simulink model "pm4_motor"  (R2017a)
settings: Solver=VariableStepAuto  StartTime=0.0  StopTime=3.0  RelTol=1e-3
libraries: simulink x1
settings Model: Creator=robotica  LastModifiedBy=robotica

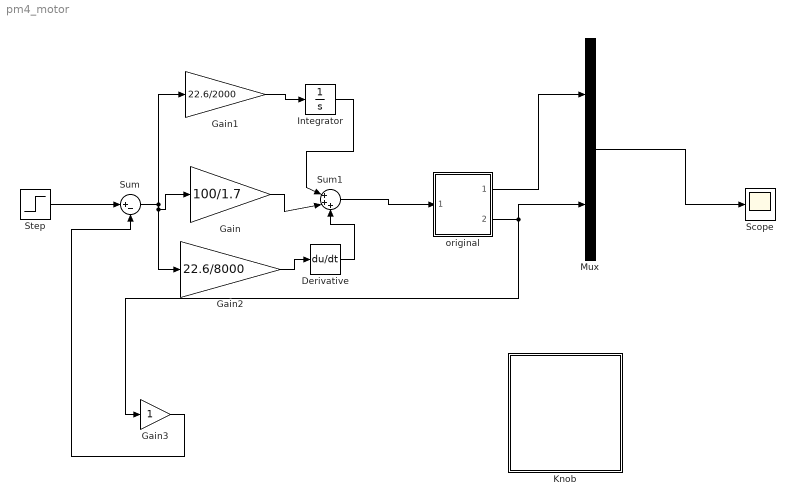
== system pm4_motor ==
  Derivative : Derivative
  Gain : Gain  Gain=100/1.7
  Gain1 : Gain  Gain=22.6/2000
  Gain2 : Gain  Gain=22.6/8000
  Gain3 : Gain
  Integrator : Integrator
  Knob : Subsystem  DialogController=hmiCreateDDGDialog  IsWebBlock=on  mask(MWDashboardBlock){webBlockId=eb4c633d-9a67-487d-a5e6-ad79ce51d936, webBlockType=continuousknob, ShowInLibBrowser=on, ShowInitialText=on, HMISrcModelName=pm4_motor}
      mask prompts: webBlockId "WebBlock Id"; webBlockType "WebBlock Type"; HMISrcModelName "Source Model"
      mask help: SimulinkHMI:dialogs:ContinuousKnobDialogDesc
      mask Help: helpview([docroot '/mapfiles/simulink.map'], 'hmi_knob')
      mask Display:
      | if strcmp(get_param(bdroot(gcb),'BlockDiagramType'), 'library')
      |     image([(matlabroot) '/toolbox/simulink/hmi/icons/ContinuousKnob.png']);
      | end
  Mux : Mux  Inputs=2
  Scope : Scope
  Step : Step  SampleTime=1
  Sum : Sum  Inputs=|+-
  Sum1 : Sum  Inputs=|+++
  original : Subsystem
  wires:
  Step/1 -> Sum/1
  Mux/1 -> Scope/1
  original/2(clean) -> Gain3/1, Mux/2
  Gain/1 -> Sum1/2
  Sum/1 -> Gain1/1, Gain2/1, Gain/1
  Integrator/1 -> Sum1/1
  Derivative/1 -> Sum1/3
  Sum1/1 -> original/1("MotoMoto ")
  Gain2/1 -> Derivative/1
  Gain1/1 -> Integrator/1
  Gain3/1 -> Sum/2
  original/1(noisy) -> Mux/1

== system pm4_motor/Knob ==

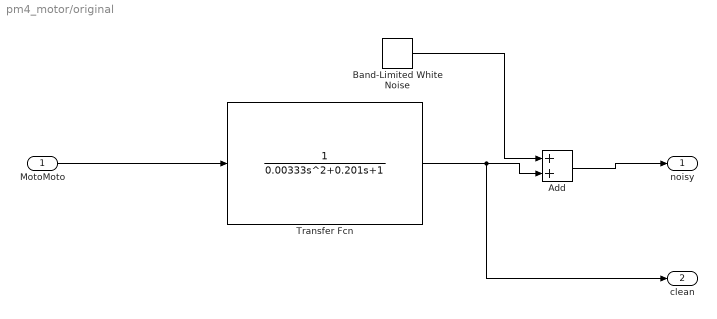
== system pm4_motor/original ==
  "MotoMoto " : Inport
  Add : Sum
  Band-Limited White Noise : simulink/Sources/Band-Limited White Noise  Cov=[0.0000001]  Ts=0.001  seed=[23341]
  Transfer Fcn : TransferFcn  Denominator=[0.00333 0.201 1]
  noisy : Outport
  clean : Outport  Port=2
  wires:
  Transfer Fcn/1 -> clean/1, Add/2
  Band-Limited White Noise/1 -> Add/1
  Add/1 -> noisy/1
  "MotoMoto "/1 -> Transfer Fcn/1
